simulink model "aquecedor_dmc"  (Simulink 7.9)
settings: Solver=ode45  StartTime=0.0  StopTime=60  FixedStep=T  RelTol=1e-3
undefined symbols (not defined in the file or in its folder): g, T
libraries: simulink x1
settings Model: Creator=Kawakami  LastModifiedBy=Kawakami
settings DataIOCC: SignalLoggingName=sigsOut
settings OptimizationCC: BooleanDataType=off
settings DebuggingCC: SaveWithParameterizedLinksMsg=none  SignalResolutionControl=TryResolveAllWithWarning  SolverPrmCheckMsg=none  MultiTaskDSMMsg=warning  MultiTaskCondExecSysMsg=none  FcnCallInpInsideContextMsg=Use local settings  StrictBusMsg=None
settings HardwareCC: TargetUnknown=on
settings RTWCC: IncludeERTFirstTime=on
settings GRTTargetCC: CombineOutputUpdateFcns=off  GRTInterface=on

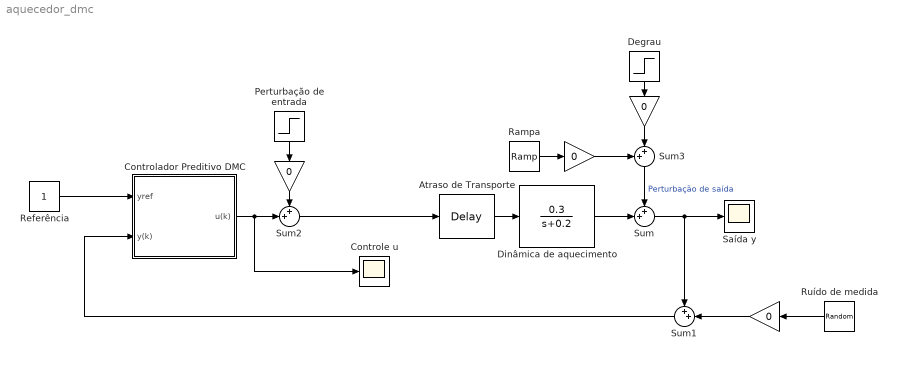
== system aquecedor_dmc ==
  " " : Gain  Gain=0
  "  " : Gain  Gain=0
  "   " : Gain  Gain=0
  "    " : Gain  Gain=0
  " Saída y" : Scope
      settings: TimeRange=60  YMin=0  YMax=1.4  SaveName=y
  Atraso de Transporte : TransportDelay  DelayTime=2
  Controlador Preditivo DMC : Subsystem  mask{rho=9.1, N=28, M=8, g=g, T=T}
      mask prompts: rho "Peso do controle (rho)"; N "Horizonte de Predição (N)"; M "Horizonte de Controle (M)"; g "Resposta a degrau da planta (g)"; T "Período de amostragem (T)"
      mask init:
      | Ns = length(g);
      | gaux = g;
      | if N > Ns
      |     gaux(Ns+1:N) = g(Ns);
      | end
      | col = gaux(1:N);
      | row = [gaux(1) zeros(1,N-1)];
      | G = toeplitz(col,row);
      | G = G(:,1:M);
      | GAIN = inv(G'*G + rho*eye(M))*G';
      | KMPC = GAIN(1,:);
  Controle u : Scope
      settings: TimeRange=60  YMin=0.2  YMax=0.9000000000000001  SaveName=u
  Degrau : Step  Time=30  After=-0.75  SampleTime=0
  Dinâmica de aquecimento : TransferFcn  Numerator=[0.3]  Denominator=[1 0.2]
  Perturbação de entrada : Step  Time=30  After=-0.5  SampleTime=0
  Rampa : simulink/Sources/Ramp  slope=-0.1  start=30  X0=0
  Referência : Constant
  Ruído de medida : RandomNumber  Variance=0.01  SampleTime=T
  Sum{,1..3} (4 alike) : Sum  Inputs=++|  SaturateOnIntegerOverflow=on  InputSameDT=on  OutDataTypeStr=Inherit: Same as first input
  wires:
  Atraso de Transporte/1 -> Dinâmica de aquecimento/1
  Dinâmica de aquecimento/1 -> Sum/2
  Sum/1 -> " Saída y"/1, Sum1/1
  Referência/1 -> Controlador Preditivo DMC/1(yref)
  Sum1/1 -> Controlador Preditivo DMC/2(y(k))
  Ruído de medida/1 -> "    "/1
  "    "/1 -> Sum1/2
  Sum2/1 -> Atraso de Transporte/1
  Controlador Preditivo DMC/1(u(k)) -> Sum2/2, Controle u/1
  Perturbação de entrada/1 -> " "/1
  " "/1 -> Sum2/1
  Degrau/1 -> "   "/1
  Rampa/1 -> "  "/1
  "  "/1 -> Sum3/1
  "   "/1 -> Sum3/2
  Sum3/1 -> Sum/1  "Perturbação de saída"

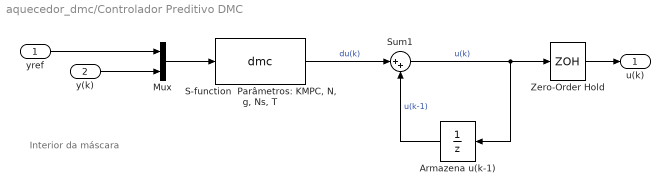
== system aquecedor_dmc/Controlador Preditivo DMC ==
  note: Interior da
      | máscara
  yref : Inport
  y(k) : Inport  Port=2
  Armazena u(k-1) : UnitDelay  SampleTime=T
  Mux : Mux  Inputs=2
  "S-function  Parâmetros: KMPC, N, g, Ns, T" : S-Function  FunctionName=dmc  Parameters=KMPC,N,g,Ns,T  EnableBusSupport=off
  Sum1 : Sum  Inputs=|++  SaturateOnIntegerOverflow=on  InputSameDT=on  OutDataTypeStr=Inherit: Same as first input
  Zero-Order Hold : ZeroOrderHold  SampleTime=T
  u(k) : Outport
  wires:
  Mux/1 -> "S-function  Parâmetros: KMPC, N, g, Ns, T"/1
  Zero-Order Hold/1 -> u(k)/1
  y(k)/1 -> Mux/2
  yref/1 -> Mux/1
  Sum1/1 -> Zero-Order Hold/1, Armazena u(k-1)/1  "u(k)"
  Armazena u(k-1)/1 -> Sum1/2  "u(k-1)"
  "S-function  Parâmetros: KMPC, N, g, Ns, T"/1 -> Sum1/1  "du(k)"
